simulink model "RobotArmSimulinkModel"  (R2017b)
settings: Solver=VariableStepAuto  StartTime=0.0  StopTime=2  RelTol=1e-3
libraries: sm_lib x14, nesl_utility x8, simulink x4
settings Model: Creator=Andrew  LastModifiedBy=Andrew

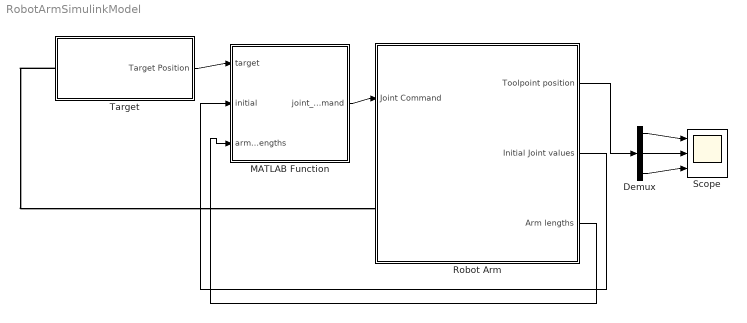
== system RobotArmSimulinkModel ==
  Demux : Demux  Outputs=3
  MATLAB Function : MATLAB Function  TreatAsAtomicUnit=on
  Robot Arm : Subsystem  mask(Robot arm simulator){q1=0, q2=0, q3=0, q4=0, lo=50, l1=100, l2=100, l3=50}
      mask prompts: q1 "initial q1 value"; q2 "initial q2 value"; q3 "initial q3 value"; q4 "initial q4 value"; lo "segment lo"; l1 "segment l1"; l2 "segment l2"; l3 "segment l3"
      mask help: Uses the simmechanics toolbox blocks and joints to make a RRRR type of robot arm. You can edit the initial joint angles in degrees and adjust the lengths of each arm segment.
      mask Help: Use the bottom left corner arrow to see how this subsystem is made
  Scope : Scope  NumInputPorts=3
  Target : Subsystem  mask(Target Block){X=150, Y=150, Z=100, a=-30}
      mask prompts: X "Target's X position"; Y "Target's Y position"; Z "Target's Z position"; a "Pitch angle"
      mask help: Edit the desired target position XYZ (in mm) and the pitch angle (in degrees) for the solver to control the robot arm. This block also spawns in the target in the simulator.
      mask Help: Use the bottom left corner arrow to see how this subsystem is made
  wires:
  Demux/1 -> Scope/1
  Demux/2 -> Scope/2
  Demux/3 -> Scope/3
  Robot Arm/1(Toolpoint position) -> Demux/1
  MATLAB Function/1(joint_command) -> Robot Arm/1(Joint Command)
  Target/1(Target Position) -> MATLAB Function/1(target)
  Robot Arm/2(Initial Joint values) -> MATLAB Function/2(initial)
  Robot Arm/3(Arm lengths) -> MATLAB Function/3(arm_lengths)
  connections:
  Target/LConn1 -- Robot Arm/LConn1

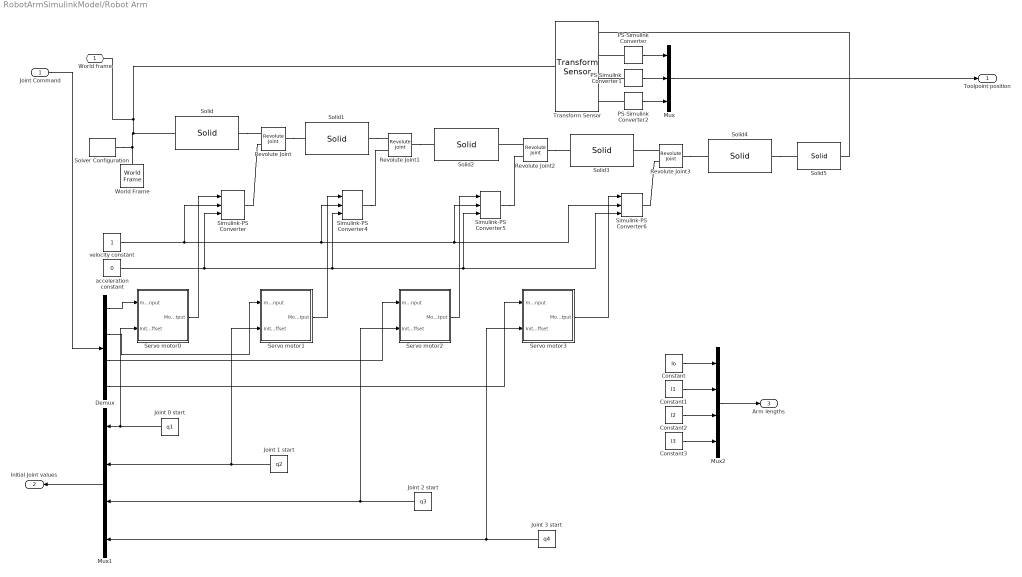
== system RobotArmSimulinkModel/Robot Arm ==
  Joint Command : Inport
  Constant : Constant  Value=lo
  Constant1 : Constant  Value=l1
  Constant2 : Constant  Value=l2
  Constant3 : Constant  Value=l3
  Demux : Demux
  Joint 0 start : Constant  Value=q1
  Joint 1 start : Constant  Value=q2
  Joint 2 start : Constant  Value=q3
  Joint 3 start : Constant  Value=q4
  Mux : Mux  Inputs=3
  Mux1 : Mux
  Mux2 : Mux
  PS-Simulink Converter : nesl_utility/PS-Simulink Converter  PhysicalDomain=network_engine_domain  SubClassName=ps_output  LeftPortType=input  RightPortType=output  PseudoPeriodic=off  Frequencies=[]  Unit=1  AffineConversion=off
  PS-Simulink Converter1 : nesl_utility/PS-Simulink Converter  PhysicalDomain=network_engine_domain  SubClassName=ps_output  LeftPortType=input  RightPortType=output  PseudoPeriodic=off  Frequencies=[]  Unit=1  AffineConversion=off
  PS-Simulink Converter2 : nesl_utility/PS-Simulink Converter  PhysicalDomain=network_engine_domain  SubClassName=ps_output  LeftPortType=input  RightPortType=output  PseudoPeriodic=off  Frequencies=[]  Unit=1  AffineConversion=off
  Revolute Joint{,1..3} (4 alike) : sm_lib/Joints/Revolute Joint  SenseConstraintForce=off  SenseConstraintForceX=off  SenseConstraintForceY=off  SenseConstraintForceZ=off  SenseConstraintTorque=off  SenseConstraintTorqueX=off  SenseConstraintTorqueY=off  SenseConstraintTorqueZ=off  SenseTotalForce=off  SenseTotalForceX=off  SenseTotalForceY=off  SenseTotalForceZ=off  SenseTotalTorque=off  SenseTotalTorqueX=off  SenseTotalTorqueY=off  SenseTotalTorqueZ=off  CompositeWrenchDir=FollowerOnBase  CompositeWrenchFrame=BaseFrame  EquilibriumPosition=0  EquilibriumPositionUnits=deg  SpringStiffness=0  SpringStiffnessUnits=N*m/deg  DampingCoefficient=0  DampingCoefficientUnits=N*m/(deg/s)  TorqueActuationMode=ComputedTorque  MotionActuationMode=InputMotion  SensePosition=off  SenseVelocity=off  SenseAcceleration=off  SenseTorqueForce=off  PositionTargetSpecify=off  PositionTargetPriority=High  PositionTargetValue=0  PositionTargetValueUnits=deg  VelocityTargetSpecify=off  VelocityTargetPriority=High  VelocityTargetValue=0  VelocityTargetValueUnits=deg/s
  Servo motor0 : Subsystem
  Servo motor1 : Subsystem
  Servo motor2 : Subsystem
  Servo motor3 : Subsystem
  Simulink-PS Converter{,4..6} (4 alike) : nesl_utility/Simulink-PS Converter  PhysicalDomain=network_engine_domain  SubClassName=ps_input  LeftPortType=input  RightPortType=output  PseudoPeriodic=off  Frequencies=[]  NoiseDistribution=none  NoiseParameters=[]  Unit=rad  AffineConversion=off  FilteringAndDerivatives=provide  SimscapeFilterOrder=1  InputFilterTimeConstant=0.001  UdotUserProvided=2
  Solid : sm_lib/Body Elements/Solid  InertiaType=CalculateFromGeometry  Mass=1  MassUnits=kg  CenterOfMass=[0 0 0]  CenterOfMassUnits=m  MomentsOfInertia=[1 1 1]  MomentsOfInertiaUnits=kg*m^2  ProductsOfInertia=[1 1 1]  ProductsOfInertiaUnits=kg*m^2  DensityBased=on  Density=1000  DensityUnits=kg/m^3  DoExposeReferenceFrame=off  SerializedFrames=<Frames><Frame><Id>Frame1</Id><Value><Name>Joint0</Name><Origin><Source>GeometricFeature</Source><FeatureName>top surface</FeatureName></Origin><PrimaryAxis><DefinedDirection>+Z</DefinedDirection><Source>ReferenceFrame</Source><SourceDirection>+Z</SourceDirection><FeatureName></FeatureName></PrimaryAxis><SecondaryAxis><DefinedDirection>+X</DefinedDirection><Source>ReferenceFrame</Source><SourceDirection>+X</SourceDirection><FeatureName></FeatureName></SecondaryAxis></Value></Frame><Frame><Id>Frame2</Id><Value><Name>Base</Name><Origin><Source>GeometricFeature</Source><FeatureName>bottom surface</FeatureName></Origin><PrimaryAxis><DefinedDirection>+Z</DefinedDirection><Source>ReferenceFrame</Source><SourceDirection>+Z</SourceDirection><FeatureName></FeatureName></PrimaryAxis><SecondaryAxis><DefinedDirection>+X</DefinedDirection><Source>ReferenceFrame</Source><SourceDirection>+X</SourceDirection><FeatureName></FeatureName></SecondaryAxis></Value></Frame></Frames>  GraphicType=FromGeometry  MarkerShape=Sphere  MarkerSize=10  GraphicVisPropType=SimpleVisualProperties  GraphicDiffuseColor=[0.5 0.5 0.5]  GraphicSpecularColor=[0.5 0.5 0.5 1.0]  GraphicAmbientColor=[0.15 0.15 0.15 1.0]  GraphicEmissiveColor=[0.0 0.0 0.0 1.0]  GraphicShininess=75  GraphicOpacity=1.0  GeometryShape=Cylinder  RectangleSize=[1 1]  RectangleSizeUnits=m  BrickDimensions=[1 1 1]  BrickDimensionUnits=m  CylinderRadius=50  CylinderRadiusUnits=mm  CylinderLength=(lo/2)  CylinderLengthUnits=mm  SphereRadius=1  SphereRadiusUnits=m  EllipsoidRadii=[1 1 1]  EllipsoidRadiiUnits=m  ExtrusionCrossSection=[1 1; -1 1; -1 -1; 1 -1]  ExtrusionCrossSectionUnits=m  ExtrusionLength=1  ExtrusionLengthUnits=m  PolygonNumSides=3  PolygonOuterRadius=1  PolygonOuterRadiusUnits=m  ExtGeomFileType=STEP  ExtGeomFileUnits=m  RevolutionCrossSection=[1 1; 1 -1; 2 -1; 2 1]  RevolutionCrossSectionUnits=m  RevolutionExtent=Full  RevolutionAngle=180  RevolutionAngleUnits=deg
  Solid1 : sm_lib/Body Elements/Solid  InertiaType=CalculateFromGeometry  Mass=1  MassUnits=kg  CenterOfMass=[0 0 0]  CenterOfMassUnits=m  MomentsOfInertia=[1 1 1]  MomentsOfInertiaUnits=kg*m^2  ProductsOfInertia=[1 1 1]  ProductsOfInertiaUnits=kg*m^2  DensityBased=on  Density=1000  DensityUnits=kg/m^3  DoExposeReferenceFrame=off  SerializedFrames=<Frames><Frame><Id>Frame1</Id><Value><Name>Joint1</Name><Origin><Source>GeometricFeature</Source><FeatureName>top surface</FeatureName></Origin><PrimaryAxis><DefinedDirection>-X</DefinedDirection><Source>ReferenceFrame</Source><SourceDirection>+Z</SourceDirection><FeatureName></FeatureName></PrimaryAxis><SecondaryAxis><DefinedDirection>+Y</DefinedDirection><Source>ReferenceFrame</Source><SourceDirection>+X</SourceDirection><FeatureName></FeatureName></SecondaryAxis></Value></Frame><Frame><Id>Frame2</Id><Value><Name>Joint0</Name><Origin><Source>GeometricFeature</Source><FeatureName>bottom curve</FeatureName></Origin><PrimaryAxis><DefinedDirection>+Z</DefinedDirection><Source>ReferenceFrame</Source><SourceDirection>+Z</SourceDirection><FeatureName></FeatureName></PrimaryAxis><SecondaryAxis><DefinedDirection>+X</DefinedDirection><Source>ReferenceFrame</Source><SourceDirection>+X</SourceDirection><FeatureName></FeatureName></SecondaryAxis></Value></Frame></Frames>  GraphicType=FromGeometry  MarkerShape=Sphere  MarkerSize=10  GraphicVisPropType=SimpleVisualProperties  GraphicDiffuseColor=[0.5 0.5 0.5]  GraphicSpecularColor=[0.5 0.5 0.5 1.0]  GraphicAmbientColor=[0.15 0.15 0.15 1.0]  GraphicEmissiveColor=[0.0 0.0 0.0 1.0]  GraphicShininess=75  GraphicOpacity=1.0  GeometryShape=Cylinder  RectangleSize=[1 1]  RectangleSizeUnits=m  BrickDimensions=[1 1 1]  BrickDimensionUnits=m  CylinderRadius=30  CylinderRadiusUnits=mm  CylinderLength=(lo/2)  CylinderLengthUnits=mm  SphereRadius=1  SphereRadiusUnits=m  EllipsoidRadii=[1 1 1]  EllipsoidRadiiUnits=m  ExtrusionCrossSection=[1 1; -1 1; -1 -1; 1 -1]  ExtrusionCrossSectionUnits=m  ExtrusionLength=1  ExtrusionLengthUnits=m  PolygonNumSides=3  PolygonOuterRadius=1  PolygonOuterRadiusUnits=m  ExtGeomFileType=STEP  ExtGeomFileUnits=m  RevolutionCrossSection=[1 1; 1 -1; 2 -1; 2 1]  RevolutionCrossSectionUnits=m  RevolutionExtent=Full  RevolutionAngle=180  RevolutionAngleUnits=deg
  Solid2 : sm_lib/Body Elements/Solid  InertiaType=CalculateFromGeometry  Mass=1  MassUnits=kg  CenterOfMass=[0 0 0]  CenterOfMassUnits=m  MomentsOfInertia=[1 1 1]  MomentsOfInertiaUnits=kg*m^2  ProductsOfInertia=[1 1 1]  ProductsOfInertiaUnits=kg*m^2  DensityBased=on  Density=1000  DensityUnits=kg/m^3  DoExposeReferenceFrame=off  SerializedFrames=<Frames><Frame><Id>Frame1</Id><Value><Name>Joint1</Name><Origin><Source>GeometricFeature</Source><FeatureName>-z surface</FeatureName></Origin><PrimaryAxis><DefinedDirection>+Y</DefinedDirection><Source>ReferenceFrame</Source><SourceDirection>+Z</SourceDirection><FeatureName></FeatureName></PrimaryAxis><SecondaryAxis><DefinedDirection>+X</DefinedDirection><Source>ReferenceFrame</Source><SourceDirection>+X</SourceDirection><FeatureName></FeatureName></SecondaryAxis></Value></Frame><Frame><Id>Frame2</Id><Value><Name>Joint2</Name><Origin><Source>GeometricFeature</Source><FeatureName>+z surface</FeatureName></Origin><PrimaryAxis><DefinedDirection>+Y</DefinedDirection><Source>ReferenceFrame</Source><SourceDirection>+Z</SourceDirection><FeatureName></FeatureName></PrimaryAxis><SecondaryAxis><DefinedDirection>+X</DefinedDirection><Source>ReferenceFrame</Source><SourceDirection>+X</SourceDirection><FeatureName></FeatureName></SecondaryAxis></Value></Frame></Frames>  GraphicType=FromGeometry  MarkerShape=Sphere  MarkerSize=10  GraphicVisPropType=SimpleVisualProperties  GraphicDiffuseColor=[0.5 0.5 0.5]  GraphicSpecularColor=[0.5 0.5 0.5 1.0]  GraphicAmbientColor=[0.15 0.15 0.15 1.0]  GraphicEmissiveColor=[0.0 0.0 0.0 1.0]  GraphicShininess=75  GraphicOpacity=1.0  GeometryShape=Brick  RectangleSize=[1 1]  RectangleSizeUnits=m  BrickDimensions=[25 25 l1]  BrickDimensionUnits=mm  CylinderRadius=30  CylinderRadiusUnits=mm  CylinderLength=50  CylinderLengthUnits=mm  SphereRadius=1  SphereRadiusUnits=m  EllipsoidRadii=[1 1 1]  EllipsoidRadiiUnits=m  ExtrusionCrossSection=[1 1; -1 1; -1 -1; 1 -1]  ExtrusionCrossSectionUnits=m  ExtrusionLength=1  ExtrusionLengthUnits=m  PolygonNumSides=3  PolygonOuterRadius=1  PolygonOuterRadiusUnits=m  ExtGeomFileType=STEP  ExtGeomFileUnits=m  RevolutionCrossSection=[1 1; 1 -1; 2 -1; 2 1]  RevolutionCrossSectionUnits=m  RevolutionExtent=Full  RevolutionAngle=180  RevolutionAngleUnits=deg
  Solid3 : sm_lib/Body Elements/Solid  InertiaType=CalculateFromGeometry  Mass=1  MassUnits=kg  CenterOfMass=[0 0 0]  CenterOfMassUnits=m  MomentsOfInertia=[1 1 1]  MomentsOfInertiaUnits=kg*m^2  ProductsOfInertia=[1 1 1]  ProductsOfInertiaUnits=kg*m^2  DensityBased=on  Density=1000  DensityUnits=kg/m^3  DoExposeReferenceFrame=off  SerializedFrames=<Frames><Frame><Id>Frame1</Id><Value><Name>Joint2</Name><Origin><Source>GeometricFeature</Source><FeatureName>-x surface</FeatureName></Origin><PrimaryAxis><DefinedDirection>-X</DefinedDirection><Source>ReferenceFrame</Source><SourceDirection>+Z</SourceDirection><FeatureName></FeatureName></PrimaryAxis><SecondaryAxis><DefinedDirection>+Y</DefinedDirection><Source>ReferenceFrame</Source><SourceDirection>+X</SourceDirection><FeatureName></FeatureName></SecondaryAxis></Value></Frame><Frame><Id>Frame2</Id><Value><Name>Joint3</Name><Origin><Source>GeometricFeature</Source><FeatureName>+x surface</FeatureName></Origin><PrimaryAxis><DefinedDirection>-X</DefinedDirection><Source>ReferenceFrame</Source><SourceDirection>+Z</SourceDirection><FeatureName></FeatureName></PrimaryAxis><SecondaryAxis><DefinedDirection>+Y</DefinedDirection><Source>ReferenceFrame</Source><SourceDirection>+X</SourceDirection><FeatureName></FeatureName></SecondaryAxis></Value></Frame></Frames>  GraphicType=FromGeometry  MarkerShape=Sphere  MarkerSize=10  GraphicVisPropType=SimpleVisualProperties  GraphicDiffuseColor=[0.5 0.5 0.5]  GraphicSpecularColor=[0.5 0.5 0.5 1.0]  GraphicAmbientColor=[0.15 0.15 0.15 1.0]  GraphicEmissiveColor=[0.0 0.0 0.0 1.0]  GraphicShininess=75  GraphicOpacity=1.0  GeometryShape=Brick  RectangleSize=[1 1]  RectangleSizeUnits=m  BrickDimensions=[l2 25 25]  BrickDimensionUnits=mm  CylinderRadius=30  CylinderRadiusUnits=mm  CylinderLength=50  CylinderLengthUnits=mm  SphereRadius=1  SphereRadiusUnits=m  EllipsoidRadii=[1 1 1]  EllipsoidRadiiUnits=m  ExtrusionCrossSection=[1 1; -1 1; -1 -1; 1 -1]  ExtrusionCrossSectionUnits=m  ExtrusionLength=1  ExtrusionLengthUnits=m  PolygonNumSides=3  PolygonOuterRadius=1  PolygonOuterRadiusUnits=m  ExtGeomFileType=STEP  ExtGeomFileUnits=m  RevolutionCrossSection=[1 1; 1 -1; 2 -1; 2 1]  RevolutionCrossSectionUnits=m  RevolutionExtent=Full  RevolutionAngle=180  RevolutionAngleUnits=deg
  Solid4 : sm_lib/Body Elements/Solid  InertiaType=CalculateFromGeometry  Mass=1  MassUnits=kg  CenterOfMass=[0 0 0]  CenterOfMassUnits=m  MomentsOfInertia=[1 1 1]  MomentsOfInertiaUnits=kg*m^2  ProductsOfInertia=[1 1 1]  ProductsOfInertiaUnits=kg*m^2  DensityBased=on  Density=1000  DensityUnits=kg/m^3  DoExposeReferenceFrame=off  SerializedFrames=<Frames><Frame><Id>Frame1</Id><Value><Name>Endeffector</Name><Origin><Source>GeometricFeature</Source><FeatureName>+z surface</FeatureName></Origin><PrimaryAxis><DefinedDirection>+Y</DefinedDirection><Source>ReferenceFrame</Source><SourceDirection>+Z</SourceDirection><FeatureName></FeatureName></PrimaryAxis><SecondaryAxis><DefinedDirection>+X</DefinedDirection><Source>ReferenceFrame</Source><SourceDirection>+X</SourceDirection><FeatureName></FeatureName></SecondaryAxis></Value></Frame><Frame><Id>Frame2</Id><Value><Name>Joint3</Name><Origin><Source>GeometricFeature</Source><FeatureName>-z surface</FeatureName></Origin><PrimaryAxis><DefinedDirection>+Y</DefinedDirection><Source>ReferenceFrame</Source><SourceDirection>+Z</SourceDirection><FeatureName></FeatureName></PrimaryAxis><SecondaryAxis><DefinedDirection>+X</DefinedDirection><Source>ReferenceFrame</Source><SourceDirection>+X</SourceDirection><FeatureName></FeatureName></SecondaryAxis></Value></Frame></Frames>  GraphicType=FromGeometry  MarkerShape=Sphere  MarkerSize=10  GraphicVisPropType=SimpleVisualProperties  GraphicDiffuseColor=[0.5 0.5 0.5]  GraphicSpecularColor=[0.5 0.5 0.5 1.0]  GraphicAmbientColor=[0.15 0.15 0.15 1.0]  GraphicEmissiveColor=[0.0 0.0 0.0 1.0]  GraphicShininess=75  GraphicOpacity=1.0  GeometryShape=Brick  RectangleSize=[1 1]  RectangleSizeUnits=m  BrickDimensions=[25 25 (l3-30)]  BrickDimensionUnits=mm  CylinderRadius=30  CylinderRadiusUnits=mm  CylinderLength=50  CylinderLengthUnits=mm  SphereRadius=1  SphereRadiusUnits=m  EllipsoidRadii=[1 1 1]  EllipsoidRadiiUnits=m  ExtrusionCrossSection=[1 1; -1 1; -1 -1; 1 -1]  ExtrusionCrossSectionUnits=m  ExtrusionLength=1  ExtrusionLengthUnits=m  PolygonNumSides=3  PolygonOuterRadius=1  PolygonOuterRadiusUnits=m  ExtGeomFileType=STEP  ExtGeomFileUnits=m  RevolutionCrossSection=[1 1; 1 -1; 2 -1; 2 1]  RevolutionCrossSectionUnits=m  RevolutionExtent=Full  RevolutionAngle=180  RevolutionAngleUnits=deg
  Solid5 : sm_lib/Body Elements/Solid  InertiaType=CalculateFromGeometry  Mass=1  MassUnits=kg  CenterOfMass=[0 0 0]  CenterOfMassUnits=m  MomentsOfInertia=[1 1 1]  MomentsOfInertiaUnits=kg*m^2  ProductsOfInertia=[1 1 1]  ProductsOfInertiaUnits=kg*m^2  DensityBased=on  Density=1000  DensityUnits=kg/m^3  DoExposeReferenceFrame=on  SerializedFrames=<Frames><Frame><Id>Frame1</Id><Value><Name>Endeffector</Name><Origin><Source>ReferenceFrame</Source><FeatureName></FeatureName></Origin><PrimaryAxis><DefinedDirection>+X</DefinedDirection><Source>ReferenceFrame</Source><SourceDirection>-Z</SourceDirection><FeatureName></FeatureName></PrimaryAxis><SecondaryAxis><DefinedDirection>+Z</DefinedDirection><Source>ReferenceFrame</Source><SourceDirection>+X</SourceDirection><FeatureName></FeatureName></SecondaryAxis></Value></Frame></Frames>  GraphicType=FromGeometry  MarkerShape=Sphere  MarkerSize=10  GraphicVisPropType=SimpleVisualProperties  GraphicDiffuseColor=[0.5 0.5 0.5]  GraphicSpecularColor=[0.5 0.5 0.5 1.0]  GraphicAmbientColor=[0.15 0.15 0.15 1.0]  GraphicEmissiveColor=[0.0 0.0 0.0 1.0]  GraphicShininess=75  GraphicOpacity=1.0  GeometryShape=GeneralExtrusion  RectangleSize=[1 1]  RectangleSizeUnits=m  BrickDimensions=[1 1 1]  BrickDimensionUnits=m  CylinderRadius=1  CylinderRadiusUnits=m  CylinderLength=1  CylinderLengthUnits=m  SphereRadius=1  SphereRadiusUnits=m  EllipsoidRadii=[1 1 1]  EllipsoidRadiiUnits=m  ExtrusionCrossSection=[2 0; 2 2; 1 3; 1 1; -1 1; -1 3; -2 2; -2 0]  ExtrusionCrossSectionUnits=cm  ExtrusionLength=25  ExtrusionLengthUnits=mm  PolygonNumSides=3  PolygonOuterRadius=1  PolygonOuterRadiusUnits=m  ExtGeomFileType=STEP  ExtGeomFileUnits=m  RevolutionCrossSection=[1 1; 1 -1; 2 -1; 2 1]  RevolutionCrossSectionUnits=m  RevolutionExtent=Full  RevolutionAngle=180  RevolutionAngleUnits=deg
  Solver Configuration : nesl_utility/Solver Configuration  PhysicalDomain=network_engine_domain  SubClassName=solver  LeftPortType=input  RightPortType=generic  Accelerate=off  Tones=[]  Harmonics=[]  SimulateNoise=off  Profile=off  UseLocalSampling=off  EnableSwitchedLinearOptims=on  FrequencyDomain=off  UseCCode=off  RelTol=0.001  AbsTol=1e-06  MinStep=1e-09  ToWorkspace=off  RevertToSquareIcSolve=off  NumHomotopyIterations=100  PhasorMode=off  PhasorModeNumHarmonics=1  DoDC=off  ResidualTolerance=1e-09  UseLocalSolver=off  LocalSolverChoice=NE_BACKWARD_EULER_ADVANCER  LocalSolverSampleTime=0.001  DoFixedCost=off  MaxNonlinIter=3  MaxModeIter=2  LinearAlgebra=Sparse  DelaysMemoryBudget=1024  AutomaticFiltering=on  FilteringTimeConstant=0.001
  Transform Sensor : sm_lib/Frames and Transforms/Transform Sensor  MeasurementFrame=World  SenseAngle=off  SenseAxis=off  SenseAngle1=off  SenseAngle2=off  SenseAngle3=off  SenseQ=off  SenseR=off  SenseOmegaX=off  SenseOmegaY=off  SenseOmegaZ=off  SenseOmega1=off  SenseOmega2=off  SenseOmega3=off  SenseQDot=off  SenseRDot=off  SenseAlphaX=off  SenseAlphaY=off  SenseAlphaZ=off  SenseAlpha1=off  SenseAlpha2=off  SenseAlpha3=off  SenseQDDot=off  SenseRDDot=off  SenseX=on  SenseY=on  SenseZ=on  SenseRad=off  SenseAzim=off  SenseDist=off  SenseInc=off  SenseXDot=off  SenseYDot=off  SenseZDot=off  SenseRadDot=off  SenseAzimDot=off  SenseDistDot=off  SenseIncDot=off  SenseXDDot=off  SenseYDDot=off  SenseZDDot=off  SenseRadDDot=off  SenseAzimDDot=off  SenseDistDDot=off  SenseIncDDot=off
  World Frame : sm_lib/Frames and Transforms/World Frame
  acceleration constant : Constant  Value=0
  velocity constant : Constant
  World frame : PMIOPort  Port=1  Side=Left
  Toolpoint position : Outport
  Initial Joint values : Outport  Port=2
  Arm lengths : Outport  Port=3
  wires:
  Joint Command/1 -> Demux/1
  PS-Simulink Converter/1 -> Mux/1
  PS-Simulink Converter2/1 -> Mux/3
  PS-Simulink Converter1/1 -> Mux/2
  Mux/1 -> Toolpoint position/1
  velocity constant/1 -> Simulink-PS Converter/2, Simulink-PS Converter4/2, Simulink-PS Converter5/2, Simulink-PS Converter6/2
  acceleration constant/1 -> Simulink-PS Converter/3, Simulink-PS Converter4/3, Simulink-PS Converter5/3, Simulink-PS Converter6/3
  Servo motor0/1(Motor output) -> Simulink-PS Converter/1
  Servo motor1/1(Motor output) -> Simulink-PS Converter4/1
  Servo motor2/1(Motor output) -> Simulink-PS Converter5/1
  Servo motor3/1(Motor output) -> Simulink-PS Converter6/1
  Demux/1 -> Servo motor0/1(motor input)
  Demux/2 -> Servo motor1/1(motor input)
  Demux/3 -> Servo motor2/1(motor input)
  Demux/4 -> Servo motor3/1(motor input)
  Joint 3 start/1 -> Servo motor3/2(Initial offset), Mux1/4
  Joint 2 start/1 -> Servo motor2/2(Initial offset), Mux1/3
  Joint 0 start/1 -> Servo motor0/2(Initial offset), Mux1/1
  Joint 1 start/1 -> Servo motor1/2(Initial offset), Mux1/2
  Mux1/1 -> Initial Joint values/1
  Constant3/1 -> Mux2/4
  Constant2/1 -> Mux2/3
  Constant1/1 -> Mux2/2
  Constant/1 -> Mux2/1
  Mux2/1 -> Arm lengths/1
  connections:
  World Frame/RConn1 -- Solver Configuration/RConn1 -- World frame/RConn1 -- Transform Sensor/LConn1 -- Solid/RConn1
  Solid/LConn1 -- Revolute Joint/LConn1
  Revolute Joint/RConn1 -- Solid1/RConn1
  Solid1/LConn1 -- Revolute Joint1/LConn1
  Revolute Joint1/RConn1 -- Solid2/LConn1
  Revolute Joint2/LConn1 -- Solid2/RConn1
  Revolute Joint2/RConn1 -- Solid3/LConn1
  Revolute Joint3/LConn1 -- Solid3/RConn1
  Solid5/RConn1 -- Transform Sensor/RConn1
  PS-Simulink Converter/LConn1 -- Transform Sensor/RConn2
  PS-Simulink Converter2/LConn1 -- Transform Sensor/RConn4
  PS-Simulink Converter1/LConn1 -- Transform Sensor/RConn3
  Simulink-PS Converter/RConn1 -- Revolute Joint/LConn2
  Simulink-PS Converter4/RConn1 -- Revolute Joint1/LConn2
  Simulink-PS Converter5/RConn1 -- Revolute Joint2/LConn2
  Simulink-PS Converter6/RConn1 -- Revolute Joint3/LConn2
  Revolute Joint3/RConn1 -- Solid4/RConn1
  Solid4/LConn1 -- Solid5/LConn1

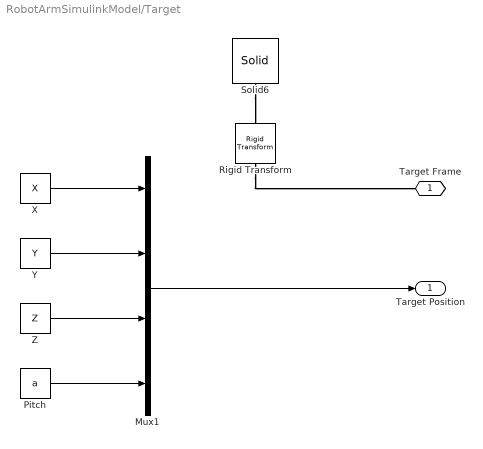
== system RobotArmSimulinkModel/Target ==
  Mux1 : Mux
  Pitch : Constant  Value=a
  Rigid Transform : sm_lib/Frames and Transforms/Rigid Transform  TranslationMethod=Cartesian  TranslationStandardOffset=0  TranslationLengthUnit=mm  TranslationStandardAxis=+Z  TranslationCartesianOffset=[X Y Z]  TranslationROffset=0  TranslationROffsetUnits=m  TranslationZOffset=0  TranslationZOffsetUnits=m  TranslationThetaOffset=0  TranslationThetaOffsetUnits=deg  RotationMethod=None  RotationAngleUnits=deg  RotationStandardAxis=+Z  RotationAngle=0.0  RotationArbitraryAxis=[0 0 1]  FollAlignAxisA=+X  BaseAlignAxisA=+Y  FollAlignAxisB=+Y  BaseAlignAxisB=+Z  RotationSequenceAxes=FollowerAxes  RotationSequence=XYX  RotationSequenceAngles=[0 0 0]  RotationSequenceAnglesUnits=deg  RotationMatrix=[1 0 0; 0 1 0; 0 0 1]
  Solid6 : sm_lib/Body Elements/Solid  InertiaType=CalculateFromGeometry  Mass=1  MassUnits=kg  CenterOfMass=[0 0 0]  CenterOfMassUnits=m  MomentsOfInertia=[1 1 1]  MomentsOfInertiaUnits=kg*m^2  ProductsOfInertia=[1 1 1]  ProductsOfInertiaUnits=kg*m^2  DensityBased=on  Density=1000  DensityUnits=kg/m^3  DoExposeReferenceFrame=off  SerializedFrames=<Frames><Frame><Id>Frame1</Id><Value><Name>Target</Name><Origin><Source>CenterOfMassFrame</Source><FeatureName></FeatureName></Origin><PrimaryAxis><DefinedDirection>+Z</DefinedDirection><Source>ReferenceFrame</Source><SourceDirection>+Z</SourceDirection><FeatureName></FeatureName></PrimaryAxis><SecondaryAxis><DefinedDirection>+X</DefinedDirection><Source>ReferenceFrame</Source><SourceDirection>+X</SourceDirection><FeatureName></FeatureName></SecondaryAxis></Value></Frame></Frames>  GraphicType=FromGeometry  MarkerShape=Sphere  MarkerSize=10  GraphicVisPropType=SimpleVisualProperties  GraphicDiffuseColor=[1.0 0.0 0.0]  GraphicSpecularColor=[0.5 0.5 0.5 1.0]  GraphicAmbientColor=[0.15 0.15 0.15 1.0]  GraphicEmissiveColor=[0.0 0.0 0.0 1.0]  GraphicShininess=75  GraphicOpacity=1.0  GeometryShape=Cylinder  RectangleSize=[1 1]  RectangleSizeUnits=m  BrickDimensions=[1 1 1]  BrickDimensionUnits=m  CylinderRadius=10  CylinderRadiusUnits=mm  CylinderLength=50  CylinderLengthUnits=mm  SphereRadius=1  SphereRadiusUnits=m  EllipsoidRadii=[1 1 1]  EllipsoidRadiiUnits=m  ExtrusionCrossSection=[1 1; -1 1; -1 -1; 1 -1]  ExtrusionCrossSectionUnits=m  ExtrusionLength=1  ExtrusionLengthUnits=m  PolygonNumSides=3  PolygonOuterRadius=1  PolygonOuterRadiusUnits=m  ExtGeomFileType=STEP  ExtGeomFileUnits=m  RevolutionCrossSection=[1 1; 1 -1; 2 -1; 2 1]  RevolutionCrossSectionUnits=m  RevolutionExtent=Full  RevolutionAngle=180  RevolutionAngleUnits=deg
  X : Constant  Value=X
  Y : Constant  Value=Y
  Z : Constant  Value=Z
  Target Frame : PMIOPort  Port=1  Side=Left
  Target Position : Outport
  wires:
  Z/1 -> Mux1/3
  Y/1 -> Mux1/2
  Mux1/1 -> Target Position/1
  Pitch/1 -> Mux1/4
  X/1 -> Mux1/1
  connections:
  Solid6/LConn1 -- Rigid Transform/RConn1
  Rigid Transform/LConn1 -- Target Frame/RConn1

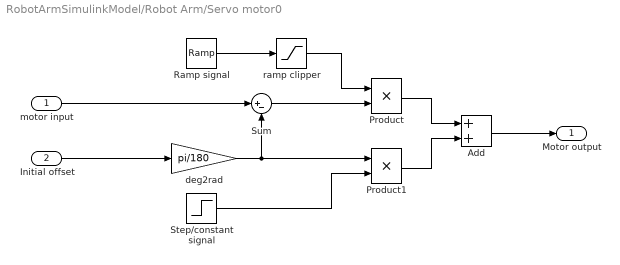
== system RobotArmSimulinkModel/Robot Arm/Servo motor0 ==
  motor input : Inport
  Initial offset : Inport  Port=2
  Add : Sum
  Product : Product
  Product1 : Product
  Ramp signal : simulink/Sources/Ramp  slope=1  start=0  X0=0
  Step/constant signal : Step  Time=0  Before=1  SampleTime=0
  Sum : Sum  Inputs=|+-
  deg2rad : Gain  Gain=pi/180
  ramp clipper : Saturate  UpperLimit=1  LowerLimit=0
  Motor output : Outport
  wires:
  ramp clipper/1 -> Product/1
  Ramp signal/1 -> ramp clipper/1
  Step/constant signal/1 -> Product1/2
  Product/1 -> Add/1
  Product1/1 -> Add/2
  Add/1 -> Motor output/1
  deg2rad/1 -> Product1/1, Sum/2
  motor input/1 -> Sum/1
  Sum/1 -> Product/2
  Initial offset/1 -> deg2rad/1

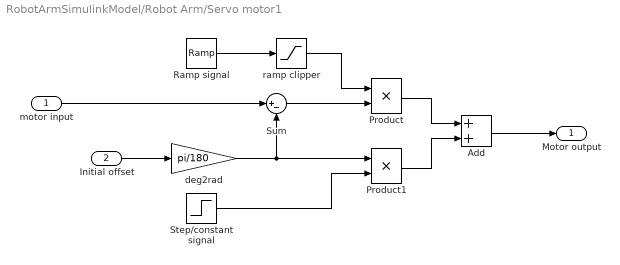
== system RobotArmSimulinkModel/Robot Arm/Servo motor1 ==
  motor input : Inport
  Initial offset : Inport  Port=2
  Add : Sum
  Product : Product
  Product1 : Product
  Ramp signal : simulink/Sources/Ramp  slope=1  start=0  X0=0
  Step/constant signal : Step  Time=0  Before=1  SampleTime=0
  Sum : Sum  Inputs=|+-
  deg2rad : Gain  Gain=pi/180
  ramp clipper : Saturate  UpperLimit=1  LowerLimit=0
  Motor output : Outport
  wires:
  ramp clipper/1 -> Product/1
  Ramp signal/1 -> ramp clipper/1
  Initial offset/1 -> deg2rad/1
  Step/constant signal/1 -> Product1/2
  Product/1 -> Add/1
  Product1/1 -> Add/2
  Add/1 -> Motor output/1
  deg2rad/1 -> Sum/2, Product1/1
  motor input/1 -> Sum/1
  Sum/1 -> Product/2

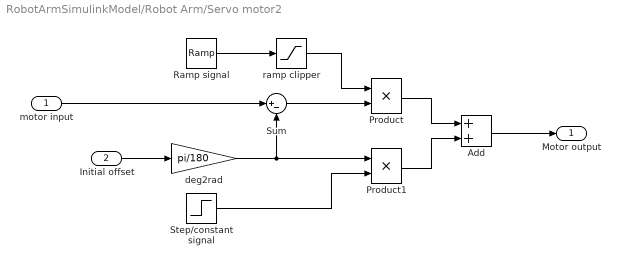
== system RobotArmSimulinkModel/Robot Arm/Servo motor2 ==
  motor input : Inport
  Initial offset : Inport  Port=2
  Add : Sum
  Product : Product
  Product1 : Product
  Ramp signal : simulink/Sources/Ramp  slope=1  start=0  X0=0
  Step/constant signal : Step  Time=0  Before=1  SampleTime=0
  Sum : Sum  Inputs=|+-
  deg2rad : Gain  Gain=pi/180
  ramp clipper : Saturate  UpperLimit=1  LowerLimit=0
  Motor output : Outport
  wires:
  ramp clipper/1 -> Product/1
  Ramp signal/1 -> ramp clipper/1
  Initial offset/1 -> deg2rad/1
  Step/constant signal/1 -> Product1/2
  Product/1 -> Add/1
  Product1/1 -> Add/2
  Add/1 -> Motor output/1
  deg2rad/1 -> Sum/2, Product1/1
  motor input/1 -> Sum/1
  Sum/1 -> Product/2

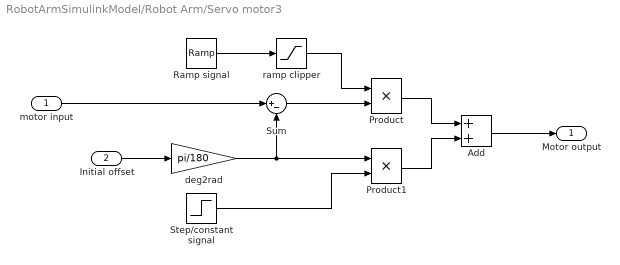
== system RobotArmSimulinkModel/Robot Arm/Servo motor3 ==
  motor input : Inport
  Initial offset : Inport  Port=2
  Add : Sum
  Product : Product
  Product1 : Product
  Ramp signal : simulink/Sources/Ramp  slope=1  start=0  X0=0
  Step/constant signal : Step  Time=0  Before=1  SampleTime=0
  Sum : Sum  Inputs=|+-
  deg2rad : Gain  Gain=pi/180
  ramp clipper : Saturate  UpperLimit=1  LowerLimit=0
  Motor output : Outport
  wires:
  ramp clipper/1 -> Product/1
  Ramp signal/1 -> ramp clipper/1
  Initial offset/1 -> deg2rad/1
  Step/constant signal/1 -> Product1/2
  Product/1 -> Add/1
  Product1/1 -> Add/2
  Add/1 -> Motor output/1
  deg2rad/1 -> Sum/2, Product1/1
  motor input/1 -> Sum/1
  Sum/1 -> Product/2

== matlab function RobotArmSimulinkModel/MATLAB Function ==
  data: target input; initial input; joint_command output; arm_lengths input
function joint_command = RobotArmController(target,initial,arm_lengths)

%Interpret Input - target and initial and arm lengths
xt = target(1);
yt = target(2);
zt = target(3);
at = -deg2rad(target(4));

q0 = deg2rad(initial(1));
q1 = deg2rad(initial(2));
q2 = deg2rad(initial(3));
q3 = deg2rad(initial(4));

lo = arm_lengths(1);
l1 = arm_lengths(2);
l2 = arm_lengths(3);
l3 = arm_lengths(4);

%Compute Inverse Kinematics

%Loop Solver
for ii=1:500
    
    %Compute Forward Kinematics from our function
    [x,y,z,a] = forwardkinematics(q0,q1,q2,q3,lo,l1,l2,l3);
    
    %Compute Velocity (Position error)
    dx = xt - x;
    dy = yt - y;
    dz = zt - z;
    da = at - a;
    
    dX = [dx dy dz da]';
    
    %Compute Jacobian from our function
    J = Jacobian_matrix(q0,q1,q2,q3,lo,l1,l2,l3);
     
    %Compute damped least squares inverse
    %pinv_J = (J'*J + eye(4))\J';
    
    %Compute output pseudo inverse Jacobian
    dQ = pinv(J)*dX;
    
    %Update joints
    q0 = q0 + dQ(1);
    q1 = q1 + dQ(2);
    q2 = q2 + dQ(3);
    q3 = q3 + dQ(4); 
    
end


%Output solution
joint_command = [q0 -q1 -q2 -q3]';

%joint_command = deg2rad(initial);

%joint_command = deg2rad([30 30 30 30]');

end

%*********DH PARAMETERS*********%
function frame1_T_frame2 = DH_params(theta,d,a,alpha)
% Computes the transformation matrix
% based on DH parameters
% A = Rz(theta)*Tz(d)*Tx(a)*Rx(alpha)

frame1_T_frame2 = [cos(theta) -sin(theta)*cos(alpha)  sin(theta)*cos(alpha) a*cos(theta);
                   sin(theta)  cos(theta)*cos(alpha) -cos(theta)*cos(alpha) a*sin(theta);
                   0           sin(alpha)             cos(alpha)            d;
                   0           0                      0                     1];

end

%*********FORWARD KINEMATICS*******%
function [x,y,z,a] = forwardkinematics(q0,q1,q2,q3,lo,l1,l2,l3)
    
    %Compute Homogeneous Transformations
    Base_T_j0 = DH_params(q0,lo,0,-pi/2);

    j0_T_j1 = DH_params(q1,0,l1,0);

    j1_T_j2 = DH_params(q2,0,l2,0);
    
    j2_T_end = DH_params(q3,0,l3,0);

    Base_T_end = Base_T_j0 * j0_T_j1 * j1_T_j2 * j2_T_end;
    
    %Compute Forward Kinematics:
    x = Base_T_end(1,4);
    y = Base_T_end(2,4);
    z = Base_T_end(3,4);
    a = sum([q1 q2 q3]);

end

%*************JACOBIAN**********%
function J = Jacobian_matrix(q1,q2,q3,q4,~,l1,l2,l3)

J = [(l2*sin(q2 - q1 + q3))/2 - sin(q1 + q2)/2 - (l3*sin(q1 + q2 + q3 + q4))/2 + (l3*sin(q2 - q1 + q3 + q4))/2 - (l1*sin(q1 - q2))/2 - (l2*sin(q1 + q2 + q3))/2, (l1*sin(q1 - q2))/2 - (l2*sin(q2 - q1 + q3))/2 - (l3*sin(q1 + q2 + q3 + q4))/2 - (l3*sin(q2 - q1 + q3 + q4))/2 - sin(q1 + q2)/2 - (l2*sin(q1 + q2 + q3))/2, - (l2*sin(q2 - q1 + q3))/2 - (l3*sin(q1 + q2 + q3 + q4))/2 - (l3*sin(q2 - q1 + q3 + q4))/2 - (l2*sin(q1 + q2 + q3))/2, -(l3*(sin(q1 + q2 + q3 + q4) + sin(q2 - q1 + q3 + q4)))/2;
                                                                                              cos(q1)*(l2*cos(q2 + q3) + l1*cos(q2) + l3*cos(q2 + q3 + q4)),                                                                                             -sin(q1)*(l2*sin(q2 + q3) + l1*sin(q2) + l3*sin(q2 + q3 + q4)),   (l3*cos(q1 + q2 + q3 + q4))/2 - (l2*cos(q2 - q1 + q3))/2 - (l3*cos(q2 - q1 + q3 + q4))/2 + (l2*cos(q1 + q2 + q3))/2,  (l3*(cos(q1 + q2 + q3 + q4) - cos(q2 - q1 + q3 + q4)))/2;
                                                                                                                                                         0,                                                                                                      - l2*cos(q2 + q3) - l1*cos(q2) - l3*cos(q2 + q3 + q4),                                                                              - l2*cos(q2 + q3) - l3*cos(q2 + q3 + q4),                                     -l3*cos(q2 + q3 + q4);
                                                                                                                                                          0,                                                                                                                                                          1,                                                                                                                     1,                                                         1];
 
end
